simulink model "Task_D"  (R2022b)
settings: Solver=ode23t  StartTime=0.0  StopTime=20.0  MaxStep=0.02  RelTol=1e-3
undefined symbols (not defined in the file): A, A_11, A_12, A_21, A_22, absolute_encoder_counts_per_revolution, B, B_1, B_2, C, init, J_r, Jgain, K_ctr, K_I
libraries: simulink_extras x10, simulink x1
settings Model: Creator=tumisangramotlhwa  LastModifiedBy=tumisangramotlhwa

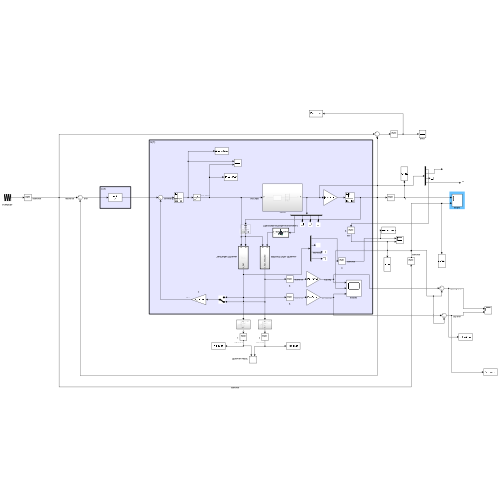
[thumbnail: Simulink's stored preview of the top-level diagram]
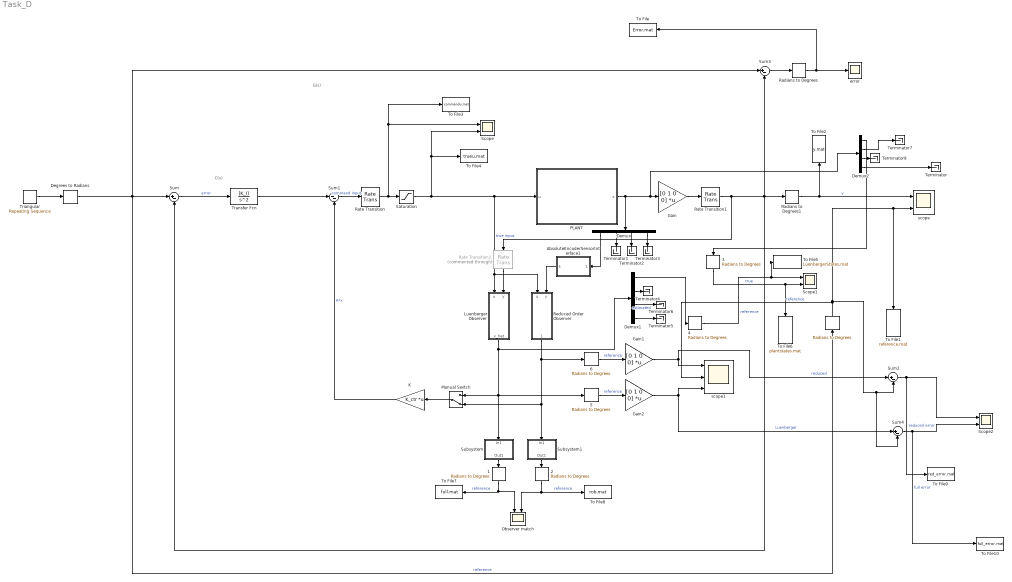
== system Task_D ==
  note: G(s)
  note: C(s)
   {,1..6} (7 alike) : simulink_extras/Transformations/Radians to Degrees
  " Triangular" : simulink/Sources/Repeating Sequence  rep_seq_t=[0 2 4]  rep_seq_y=[45 15 45]
  AbsoluteEncoderSensorInterface1 : Subsystem  TreatAsAtomicUnit=on
      mask Display: image('$imagefile'); % Use "Edit Image" on toolstrip to change.
  Degrees to Radians : simulink_extras/Transformations/Degrees to Radians
  Demux : Demux
  Demux1 : Demux
  Demux2 : Demux
  Gain : Gain  Gain=[0 1 0 0]  Multiplication=Matrix(K*u) (u vector)
  Gain1 : Gain  Gain=[0 1 0 0]  Multiplication=Matrix(K*u) (u vector)
  Gain2 : Gain  Gain=[0 1 0 0]  Multiplication=Matrix(K*u) (u vector)
  K : Gain  Gain=K_ctr  Multiplication=Matrix(K*u) (u vector)
  Luenberger Observer : Subsystem  TreatAsAtomicUnit=on
  Manual Switch : ManualSwitch  CurrentSetting=0
  Observer match : Scope  NumInputPorts=2
  PLANT : Subsystem
  Radians to Degrees : simulink_extras/Transformations/Radians to Degrees
  Radians to Degrees1 : simulink_extras/Transformations/Radians to Degrees
  Rate Transition : RateTransition  OutPortSampleTime=1/50
  Rate Transition1 : RateTransition  OutPortSampleTime=1/50
  Rate Transition2 : RateTransition  Commented=through  OutPortSampleTime=1/50
  Reduced Order Observer : Subsystem  TreatAsAtomicUnit=on
  Saturation : Saturate  UpperLimit=6  LowerLimit=-6
  Scope : Scope  NumInputPorts=2
  Scope1 : Scope  NumInputPorts=2
  Scope2 : Scope  NumInputPorts=2
  Subsystem : Subsystem
  Subsystem1 : Subsystem
  Sum{,2..4} (4 alike) : Sum  Inputs=|+-
  Sum1 : Sum  Inputs=|--
  Terminator{,1..7,9} (9 alike) : Terminator
  To File : ToFile  Filename=Error.mat  MatrixName=Error  SaveFormat=Timeseries
  To File1 : ToFile  Filename=reference.mat  MatrixName=reference  SaveFormat=Timeseries
  To File10 : ToFile  Filename=full_error.mat  MatrixName=full_error  SaveFormat=Timeseries
  To File2 : ToFile  Filename=y.mat  MatrixName=y  SaveFormat=Timeseries
  To File3 : ToFile  Filename=commandu.mat  MatrixName=commandu  SaveFormat=Timeseries
  To File4 : ToFile  Filename=trueu.mat  MatrixName=trueu  SaveFormat=Timeseries
  To File5 : ToFile  Filename=LuenbergerStates.mat  MatrixName=LuenbergerStates  SaveFormat=Timeseries
  To File6 : ToFile  Filename=plantstates.mat  MatrixName=plantstates  SaveFormat=Timeseries
  To File7 : ToFile  Filename=full.mat  MatrixName=full  SaveFormat=Timeseries
  To File8 : ToFile  Filename=rob.mat  MatrixName=rob  SaveFormat=Timeseries
  To File9 : ToFile  Filename=red_error.mat  MatrixName=red_error  SaveFormat=Timeseries
  Transfer Fcn : TransferFcn  Numerator=[K_I]  Denominator=[1 0 0]
  error : Scope
  scope : Scope  NumInputPorts=2
  scope1 : Scope  NumInputPorts=3
  wires:
  Sum/1 -> Transfer Fcn/1  "error"
  Radians to Degrees/1 -> error/1, To File/1
  Radians to Degrees1/1 -> scope/1, To File2/1  "y"
  Saturation/1 -> PLANT/1(u), Reduced Order Observer/1(u), Luenberger Observer/1(u), To File4/1, Scope/2  "true input"
  " Triangular"/1 -> Degrees to Radians/1
  Sum3/1 -> Radians to Degrees/1
  K/1 -> Sum1/2  "K*x"
  Degrees to Radians/1 -> Sum3/1, " "/1, Sum/1  "reference"
  " "/1 -> Sum4/2, Sum2/2, scope/2, To File1/1, scope1/2  "reference"
  Manual Switch/1 -> K/1
  PLANT/1(x) -> Demux2/1, Gain/1, Demux/1
  Demux/2 -> Terminator1/1
  Demux/3 -> Terminator2/1
  Demux/4 -> Terminator3/1
  " 2"/1 -> To File8/1, Observer match/2  "reference"
  " 1"/1 -> Observer match/1, To File7/1  "reference"
  Transfer Fcn/1 -> Sum1/1
  Gain/1 -> Rate Transition1/1
  Luenberger Observer/1(x_hat) -> " 5"/1, Manual Switch/1, Subsystem/1(In1), Demux1/1
  Sum1/1 -> Rate Transition/1  "command input"
  Rate Transition2/1 -> Luenberger Observer/2(y)
  Gain1/1 -> scope1/1, Sum2/1  "reduced"
  Gain2/1 -> Sum4/1, scope1/3  "Luenberger"
  " 3"/1 -> To File6/1, Scope1/2  "true"
  " 4"/1 -> To File5/1, Scope1/1  "reference"
  Demux1/1 -> " 4"/1
  Demux2/1 -> " 3"/1
  Demux2/4 -> Terminator/1
  Demux1/4 -> Terminator5/1
  Demux2/3 -> Terminator9/1
  Demux1/3 -> Terminator6/1  "estimated"
  Demux2/2 -> Terminator7/1
  Demux1/2 -> Terminator4/1
  " 5"/1 -> Gain2/1  "reference"
  " 6"/1 -> Gain1/1  "reference"
  Rate Transition/1 -> Saturation/1, To File3/1, Scope/1
  Rate Transition1/1 -> Rate Transition2/1, Sum3/2, Radians to Degrees1/1, Sum/2
  Demux/1 -> AbsoluteEncoderSensorInterface1/1(y_plant)
  Sum4/1 -> To File10/1, Scope2/2  "full error"
  Sum2/1 -> To File9/1, Scope2/1  "reduced error"
  AbsoluteEncoderSensorInterface1/1(y_absenc) -> Reduced Order Observer/2(y)
  Subsystem/1(Out1) -> " 1"/1
  Reduced Order Observer/1(x_hat_reduced) -> Subsystem1/1(In1), Manual Switch/2, " 6"/1
  Subsystem1/1(Out1) -> " 2"/1

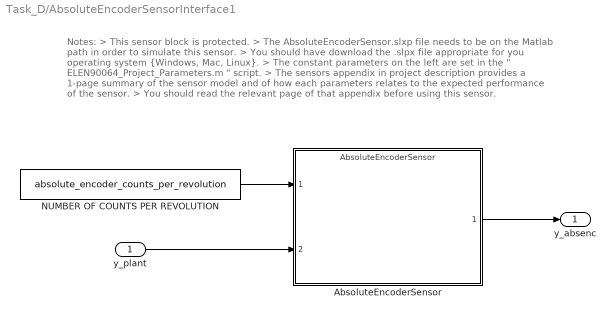
== system Task_D/AbsoluteEncoderSensorInterface1 ==
  note: Notes:
      | > This sensor block is protected.
      | > The AbsoluteEncoderSensor.slxp file needs to be on the Matlab path in order to simulate this sensor.
      | > You should have download the .slpx file appropriate for you operating system {Windows, Mac, Linux}.
      | > The constant parameters on the left are set in the " ELEN90064_Project_Parameters.m " script.
      | > The sensors appendix in project description provides a 1-page summary of the sensor model and of how each parameters relates to the expected performance of the sensor.
      | > You should read the relevant page of that appendix before using this sensor.
  y_plant : Inport
  AbsoluteEncoderSensor : ModelReference  ModelNameDialog=AbsoluteEncoderSensor.slxp  ModelReferenceVersion=1.16  CopyOfModelProtected=on
  NUMBER OF COUNTS PER REVOLUTION : Constant  Value=absolute_encoder_counts_per_revolution
  y_absenc : Outport
  wires:
  NUMBER OF COUNTS PER REVOLUTION/1 -> AbsoluteEncoderSensor/1
  y_plant/1 -> AbsoluteEncoderSensor/2
  AbsoluteEncoderSensor/1 -> y_absenc/1

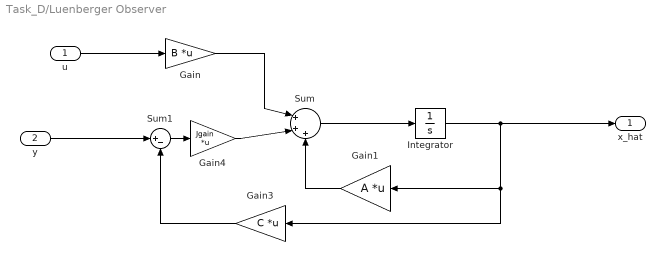
== system Task_D/Luenberger Observer ==
  u : Inport
  y : Inport  Port=2
  Gain : Gain  Gain=B  Multiplication=Matrix(K*u) (u vector)
  Gain1 : Gain  Gain=A  Multiplication=Matrix(K*u) (u vector)
  Gain3 : Gain  Gain=C  Multiplication=Matrix(K*u) (u vector)
  Gain4 : Gain  Gain=Jgain  Multiplication=Matrix(K*u) (u vector)
  Integrator : Integrator
  Sum : Sum  Inputs=|+++
  Sum1 : Sum  Inputs=|+-
  x_hat : Outport
  wires:
  Gain/1 -> Sum/1
  Gain4/1 -> Sum/2
  Sum1/1 -> Gain4/1
  Gain3/1 -> Sum1/2
  Gain1/1 -> Sum/3
  Sum/1 -> Integrator/1
  Integrator/1 -> x_hat/1, Gain1/1, Gain3/1
  u/1 -> Gain/1
  y/1 -> Sum1/1

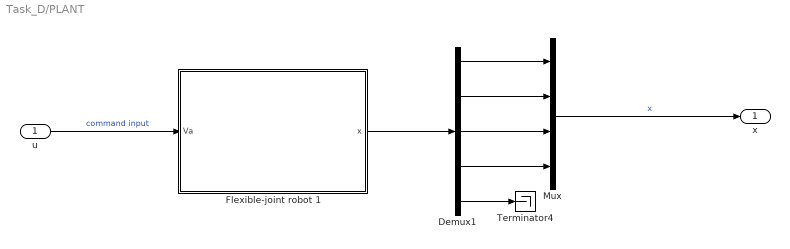
== system Task_D/PLANT ==
  u : Inport
  Demux1 : Demux  Outputs=5
  Flexible-joint robot 1 : Subsystem
      mask Display: image('$imagefile'); % Use "Edit Image" on toolstrip to change.
  Mux : Mux
  Terminator4 : Terminator
  x : Outport
  wires:
  Mux/1 -> x/1  "x"
  Demux1/4 -> Mux/4
  Flexible-joint robot 1/1(x) -> Demux1/1
  Demux1/3 -> Mux/3
  Demux1/2 -> Mux/2
  Demux1/1 -> Mux/1
  Demux1/5 -> Terminator4/1
  u/1 -> Flexible-joint robot 1/1(Va)  "command input"

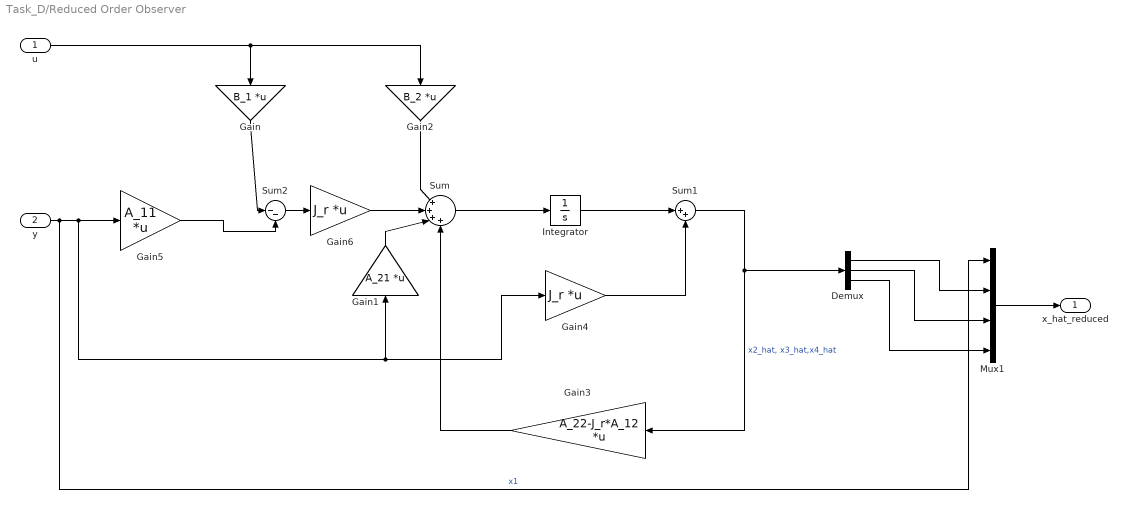
== system Task_D/Reduced Order Observer ==
  u : Inport
  y : Inport  Port=2
  Demux : Demux  Outputs=3
  Gain : Gain  Gain=B_1  Multiplication=Matrix(K*u) (u vector)
  Gain1 : Gain  Gain=A_21  Multiplication=Matrix(K*u) (u vector)
  Gain2 : Gain  Gain=B_2  Multiplication=Matrix(K*u) (u vector)
  Gain3 : Gain  Gain=A_22-J_r*A_12  Multiplication=Matrix(K*u) (u vector)
  Gain4 : Gain  Gain=J_r  Multiplication=Matrix(K*u) (u vector)
  Gain5 : Gain  Gain=A_11  Multiplication=Matrix(K*u) (u vector)
  Gain6 : Gain  Gain=J_r  Multiplication=Matrix(K*u) (u vector)
  Integrator : Integrator
  Mux1 : Mux
  Sum : Sum  Inputs=|++++
  Sum1 : Sum  Inputs=|++
  Sum2 : Sum  Inputs=|--
  x_hat_reduced : Outport
  wires:
  u/1 -> Gain2/1, Gain/1
  y/1 -> Mux1/1, Gain5/1, Gain4/1, Gain1/1  "x1"
  Sum/1 -> Integrator/1
  Gain6/1 -> Sum/2
  Gain1/1 -> Sum/3
  Gain/1 -> Sum2/1
  Gain5/1 -> Sum2/2
  Gain2/1 -> Sum/1
  Integrator/1 -> Sum1/1
  Gain4/1 -> Sum1/2
  Gain3/1 -> Sum/4
  Sum1/1 -> Demux/1, Gain3/1  "x2_hat, x3_hat,x4_hat"
  Sum2/1 -> Gain6/1
  Mux1/1 -> x_hat_reduced/1
  Demux/1 -> Mux1/2
  Demux/2 -> Mux1/3
  Demux/3 -> Mux1/4

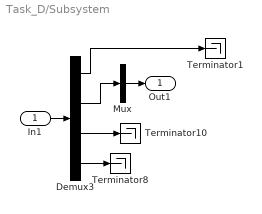
== system Task_D/Subsystem ==
  In1 : Inport
  Demux3 : Demux
  Mux : Mux  Inputs=1
  Terminator1 : Terminator
  Terminator10 : Terminator
  Terminator8 : Terminator
  Out1 : Outport
  wires:
  Mux/1 -> Out1/1
  Demux3/2 -> Mux/1
  Demux3/3 -> Terminator10/1
  In1/1 -> Demux3/1
  Demux3/4 -> Terminator8/1
  Demux3/1 -> Terminator1/1

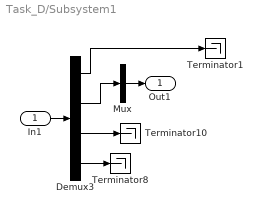
== system Task_D/Subsystem1 ==
  In1 : Inport
  Demux3 : Demux
  Mux : Mux  Inputs=1
  Terminator1 : Terminator
  Terminator10 : Terminator
  Terminator8 : Terminator
  Out1 : Outport
  wires:
  Mux/1 -> Out1/1
  Demux3/2 -> Mux/1
  Demux3/3 -> Terminator10/1
  In1/1 -> Demux3/1
  Demux3/4 -> Terminator8/1
  Demux3/1 -> Terminator1/1

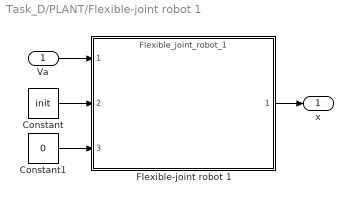
== system Task_D/PLANT/Flexible-joint robot 1 ==
  Va : Inport
  Constant : Constant  Value=init
  Constant1 : Constant  Value=0
  Flexible-joint robot 1 : ModelReference  ModelNameDialog=Flexible_joint_robot_1  ModelReferenceVersion=1.63  CopyOfModelProtected=on
  x : Outport
  wires:
  Constant/1 -> Flexible-joint robot 1/2
  Constant1/1 -> Flexible-joint robot 1/3
  Flexible-joint robot 1/1 -> x/1
  Va/1 -> Flexible-joint robot 1/1
